simulink model "SFcontrol7mod"  (Simulink 6.6)
settings: Solver=FixedStepDiscrete  StartTime=0.0  StopTime=10  FixedStep=1  RelTol=1e-3
settings Model: Creator=ksmyth  LastModifiedBy=vBuskirk
settings DebuggingCC: SignalResolutionControl=TryResolveAllWithWarning  MultiTaskDSMMsg=warning  MultiTaskCondExecSysMsg=none
settings RTWCC: IncludeERTFirstTime=on

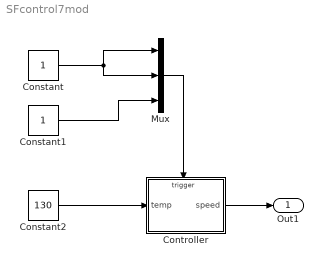
== system SFcontrol7mod ==
  Constant : Constant
  Constant1 : Constant
  Constant2 : Constant  Value=130
  Controller : Stateflow chart  TreatAsAtomicUnit=on
  Mux : Mux  Inputs=3
  Out1 : Outport
  wires:
  Mux/1 -> Controller/Trigger
  Controller/1(speed) -> Out1/1
  Constant1/1 -> Mux/3
  Constant2/1 -> Controller/1(temp)
  Constant/1 -> Mux/1, Mux/2

== stateflow chart Controller ==
  state OFF
    en:speed = 0;
  state r = hot [function]
    (default) -> (junction 10) : {r = temp >= 120;}
  state On
    (history)
    state Hi
      en:speed = 2;
    state Lo
      en:speed = 1;
    state No
      en:speed = 0;
    Hi -> Lo : [!hot()]
    Lo -> Hi [order 1] : [hot()]
    (default) -> No
    Lo -> No [order 2] : [cool()]
    No -> Lo : [!cool()]
  state r = cool [function]
    (default) -> (junction 12) : {r = temp <= 100;}
  (default) -> OFF
  OFF -> On : on_switch
  On -> OFF : off_switch
  data: r function_output boolean; r function_output boolean; speed output double; temp input inherited
  events: off_switch input FALLING_EDGE_EVENT; on_switch input RISING_EDGE_EVENT; temp_event input RISING_EDGE_EVENT
